simulink model "INDI_QUAD_2021a"  (R2026a)
settings: Solver=VariableStepAuto  StopTime=30  FixedStep=step_time
InitFcn:
  | kt = 66.34;
  | kq = 2.38;
  | M = 8.22;
  | l = 1.63/2;
  | Ix = 0.4688;
  | Iy = 0.5;
  | Iz = 0.4930;
  | g = 9.81;
  | step_time = 0.001;
  | Kz = 125;
  | Kpsi = 70;
  | Kphi = 70;
  | Ktheta = 70;
  | flt = 0.45;
undefined symbols (not defined in the file): F, Light, MIL
libraries: aerolibwind2 x1, sim3dlib x1, uavsim3dlib x1
settings Model: Creator=Lenovo  LastModifiedBy=Lenovo
settings SimscapeCC: SimscapeNominalValues="[{\"value\":\"1\",\"unit\":\"A\"},{\"value\":\"1\",\"unit\":\"bar\"},{\"value\":\"1\",\"unit\":\"cm^2\"},{\"value\":\"1\",\"unit\":\"cm^3/s\"},{\"value\":\"1\",\"unit\":\"kJ/kg\"},{\"value\":\"1\",\"unit\":\"kW\"},{\"value\":\"1\",\"unit\":\"l\"},{\"value\":\"1\",\"unit\":\"N\"},{\"value\":\"1\",\"unit\":\"N*m\"},{\"value\":\"1\",\"unit\":\"V\"}]"  SimscapeLogType=none  SimscapeLogDataHistory=5000.0

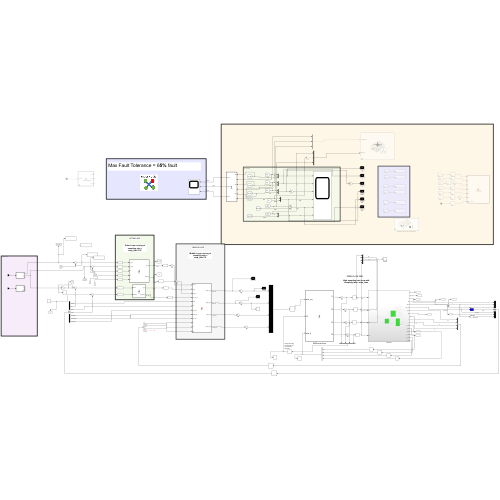
[thumbnail: Simulink's stored preview of the top-level diagram]
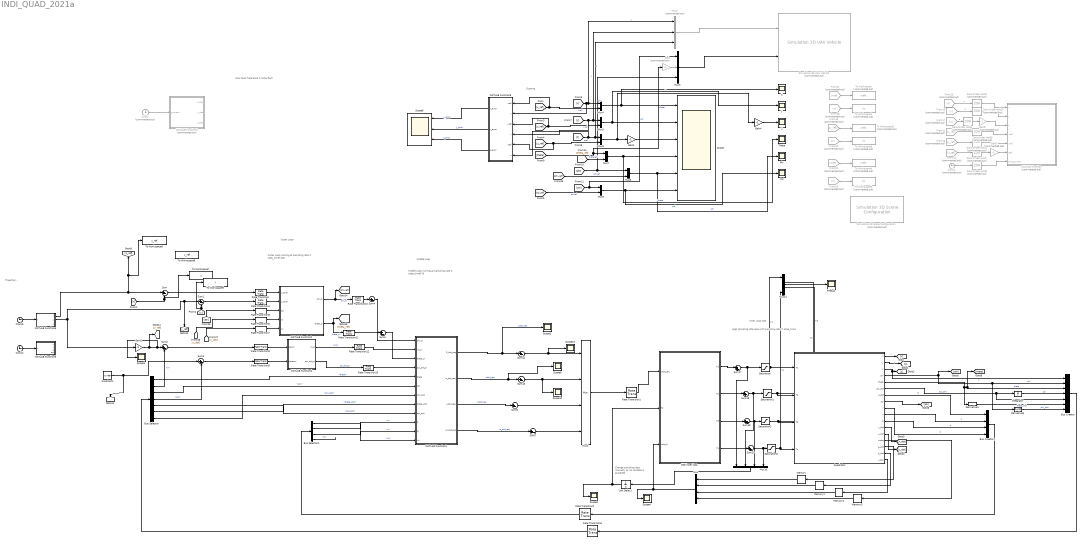
== system INDI_QUAD_2021a ==
  note: Inner Loop INDI
  note: Outer Loop
  note: Middle Loop running at sampling rate = step_time*10
  note: Trajectory
  note: Change sampling rate manually as no variable is assigned
  note: High sampling rate loop with sampling rate = step_time
  note: Max Fault Tolerance = 6 5% fault
  note: Outer Loop running at sampling rate = step_time*100
  note: Middle Loop
  note: Scoping
  Bus Creator : BusCreator  Inputs=7
  Bus Creator1 : BusCreator  Inputs=4
  Bus Selector : BusSelector  OutputSignals=theta,z,phi,psi,psi_dot,theta_dot,phi_dot
  Bus Selector1 : BusSelector  OutputSignals=Vz,p,q,R
  Clock : Clock  Commented=on
  Clock1 : Clock  Commented=on
  Clock2 : Clock
  Clock5 : Clock
  Constant1 : Constant  Value=0.7854
  Derivative1 : Derivative
  Derivative2 : Derivative
  From12 : From  Commented=on  GotoTag=x_ref
  From13 : From  Commented=on  GotoTag=y_ref
  From14 : From  Commented=on  GotoTag=z_ref
  From15 : From  Commented=on  GotoTag=x
  From16 : From  Commented=on  GotoTag=y
  From17 : From  Commented=on  GotoTag=z
  From18 : From  Commented=on  GotoTag=x
  From19 : From  Commented=on  GotoTag=y_ref
  From20 : From  Commented=on  GotoTag=zref
  From21 : From  Commented=on  GotoTag=xref
  From22 : From  Commented=on  GotoTag=y
  From23 : From  Commented=on  GotoTag=z
  Gain : Gain  Commented=on  Gain=-1
  Gain1 : Gain  Gain=-1
  Gain2 : Gain  Gain=-1
  Gain3 : Gain  Commented=on  Gain=-1
  Gain4 : Gain  Gain=-1
  Gain8 : Gain  Commented=on  Gain=-1
  INDI inner loop : MATLAB Function  TreatAsAtomicUnit=on
  Integrator : Integrator  InitialCondition=0.7854
  MATLAB Function : MATLAB Function  Commented=on  TreatAsAtomicUnit=on
  MATLAB Function1 : MATLAB Function  TreatAsAtomicUnit=on
  MATLAB Function2 : MATLAB Function  TreatAsAtomicUnit=on
  MATLAB Function3 : MATLAB Function  Commented=on  TreatAsAtomicUnit=on
  MATLAB Function4 : MATLAB Function  TreatAsAtomicUnit=on
  MATLAB Function5 : MATLAB Function  TreatAsAtomicUnit=on
  MATLAB Function6 : MATLAB Function  TreatAsAtomicUnit=on
  MATLAB Function8 : MATLAB Function  TreatAsAtomicUnit=on
  Memory{,1..3} (4 alike) : Memory
  Mux{,1,10..11} (4 alike) : Mux
  Mux2 : Mux  Commented=on  Inputs=3
  Mux3 : Mux  Inputs=3
  Mux{4..9} (6 alike) : Mux  Inputs=2
  Phi : Scope
      settings: Title=Roll angle (rad) vs Time (Seconds)  ActiveDisplayYMinimum=-0.24071  ActiveDisplayYMaximum=0.27138  YLabel=Roll angle (rad)
  Psi : Scope
      settings: Title=Yaw angle (rad) vs Time (Seconds)  ActiveDisplayYMinimum=-0.5  ActiveDisplayYMaximum=0.5  YLabel=Yaw angle (rad)  DataLoggingVariableName=ScopeData2
  Quadrotor : Subsystem
  Rate Transition{,4..9} (7 alike) : RateTransition  OutPortSampleTime=step_time*100
  Rate Transition1 : RateTransition  OutPortSampleTime=step_time
  Rate Transition{2..3,10..13} (6 alike) : RateTransition  OutPortSampleTime=step_time*10
  Saturation{,1..3} (4 alike) : Saturate  UpperLimit=1  LowerLimit=0
  Scope : Scope  NumInputPorts=6
      settings: TimeSpan=30  ActiveDisplayYMinimum=-1.4894  ActiveDisplayYMaximum=13.37546  YLabel=x(m)  DataLoggingVariableName=ScopeData3
  Scope{1..4,9,12..13} (7 alike) : Scope
      Scope1 settings: ActiveDisplayYMinimum=-11.25  ActiveDisplayYMaximum=1.25  DataLoggingVariableName=ScopeData3
      Scope12 settings: ActiveDisplayYMinimum=-0.77126  ActiveDisplayYMaximum=1.00462  DataLoggingVariableName=ScopeData5
      Scope13 settings: ActiveDisplayYMinimum=-0.61483  ActiveDisplayYMaximum=0.4623  DataLoggingVariableName=ScopeData6
      Scope2 settings: ActiveDisplayYMinimum=-0.24056  ActiveDisplayYMaximum=0.09054
      Scope3 settings: ActiveDisplayYMinimum=-0.1115  ActiveDisplayYMaximum=1.0035  DataLoggingVariableName=ScopeData5
      Scope4 settings: ActiveDisplayYMinimum=-8.06418  ActiveDisplayYMaximum=11.79602  DataLoggingVariableName=ScopeData6
      Scope9 settings: ActiveDisplayYMinimum=-0.58145  ActiveDisplayYMaximum=0.65087  DataLoggingVariableName=ScopeData2
  Scope6 : Scope  NumInputPorts=3
      settings: ActiveDisplayYMinimum=-0.92421  ActiveDisplayYMaximum=8.31793
  Simulation 3D Scene Configuration : sim3dlib/Simulation 3D Scene Configuration  Priority=0  Commented=on  ProjectFormat=Unreal Executable  SceneDesc=US city block  ProjectName=C:\Program Files\MATLAB\R2024a\toolbox\shared\sim3d_projects\automotive_project_windows\UE\WindowsNoEditor\VehicleSimulation.exe  ScenePath=/Game/Maps/USCityBlock  EnableOpenDRIVE=off  vehTagList={'Scene Origin'}  vehTag=Scene Origin  AttachedCameraRelativeTranslation=[0 0 0]  FreeCameraDefaultInitialTranslation=[-6, 0, 2]  AttachedCameraRelativeRotation=[0, -15, 0]  FreeCameraDefaultInitialRotation=[0, -15, 0]  ViewpointName=Custom  FreeCameraInitialTranslation=[0, 0, 0]  FreeCameraInitialRotation=[0, 0, 0]  OpVisEn=off  Ts=step_time*10  EnableWindow=on  EnableRemoteAccess=off  SimulationMode=CoSimulation  SimulateUsing=Interpreted execution  EnableAnimationRecording=off  OverrideDefaultRecording=off  AnimationRecordingFileName=sim3dAnimation.mat  AnimationRecordingInterval=[0 inf]  EnableWeather=off  SunAzimuth=90  SunAltitude=40.0  EnableGeospatialSun=off  Latitude=0  Longitude=0  Date=2023-01-01  Time=10:30:00  GeoTimeZone=-5.0  SunDaylightSaving=off  wind=1  clouds=10  EnableVolumetricClouds=off  CloudCoverage=0  CloudAltitude=6  fog=0  rain=0  RaindropsEffect=off  SnowDensity=0  EnableGeospatial=off  TilesetSource=Earth terrain  UseTrueOrigin=off  OriginHeight=200  OriginLatitude=40.744652  OriginLongitude=-73.988864  MapStyle=Aerial  AdditionalAssetIDs=[]  UseAdvancedSunSky=off  SolarTime=11  TimeZone=-5  Day=21  Month=9  Year=2022  UseDaylightSavingTime=on  DSTStartDay=10  DSTStartMonth=3  DSTEndDay=3  DSTEndMonth=11  DSTSwitchHour=2  sensorTag=MainCamera1  sensorId=1  sensorName=MainCamera1  mountLoc=Origin  offsetFlag=off  tmountOffset=[0, 0, 0]  rmountOffset=[0, 0, 0]  HorizontalResolution=1280  VerticalResolution=720  HorizontalFOV=60  mountPoint=[0 0 0]  mountOrientation=[0 0 0]  aMode=4  ID=1  GeoTrigger=Inactive  ViewNameList={'Custom'}  ViewTranslationList={'[0 0 0]'}  ViewRotationList={'[0 0 0]'}
      settings: LibrarySourceBlock=uavsim3dlib/Simulation 3D Scene Configuration
  Simulation 3D UAV Vehicle : uavsim3dlib/Simulation 3D UAV Vehicle  Priority=-1  Commented=on  Mesh=Quadrotor  MeshPath=/MathWorksUAVContent/UAVs/HexaRotorUAV/HexaRotor.HexaRotor  Color=Black  ActorName=SimulinkVehicle1  UseGlobalFrame=off  InitialTranslation=[0 0 0]  InitialRotation=[0 0 0]  InitialTranslationGlobal=[0 0 0]  InitialGeoOrigin=[0 0 0]  InitialRotationGlobal=[0 0 0]  SampleTime=-1  ActorType=SimulinkVehicle  ID=1  aMode=4  ActorTag=SimulinkVehicle1
  Sum{,1..7,13..14} (10 alike) : Sum  Inputs=|+-
  Sum{17..20} (4 alike) : Sum  Inputs=|++
  THeta : Scope
      settings: Title=Pitch angle (rad) vs Time (Seconds)  ActiveDisplayYMinimum=-0.27265  ActiveDisplayYMaximum=0.23706  YLabel=Pitch angle (rad)  DataLoggingVariableName=ScopeData4
  THeta1 : Scope
      settings: Title=Normalized Thrust Force vs Time (seconds)  ActiveDisplayYMinimum=-0.11657  ActiveDisplayYMaximum=1.04914  YLabel=Normalized Thrust Force  DataLoggingVariableName=ScopeData2
  To Workspace : ToWorkspace  Commented=on  VariableName=xreflc  SampleTime=-1
  To Workspace1 : ToWorkspace  Commented=on  VariableName=xlc  SampleTime=-1
  To Workspace2 : ToWorkspace  Commented=on  VariableName=yreflc  SampleTime=-1
  To Workspace3 : ToWorkspace  Commented=on  VariableName=ylc  SampleTime=-1
  To Workspace4 : ToWorkspace  Commented=on  VariableName=zreflc  SampleTime=-1
  To Workspace5 : ToWorkspace  Commented=on  VariableName=zlc  SampleTime=-1
  To Workspace6 : ToWorkspace  VariableName=x_ref  SaveFormat=Timeseries  SampleTime=-1
  To Workspace7 : ToWorkspace  VariableName=x  SaveFormat=Timeseries  SampleTime=-1
  To Workspace8 : ToWorkspace  VariableName=y_ref  SaveFormat=Timeseries  SampleTime=-1
  To Workspace9 : ToWorkspace  VariableName=y  SaveFormat=Timeseries  SampleTime=-1
  Unit Delay1 : UnitDelay  SampleTime=step_time
  X : Scope
      settings: Title=x (m) vs Time (Seconds)  ActiveDisplayYMinimum=-1.43359  ActiveDisplayYMaximum=12.90232  YLabel=X(m)  DataLoggingVariableName=ScopeData5
  Y : Scope
      settings: Title=y (m) vs Time (Seconds)  ActiveDisplayYMinimum=-1.44356  ActiveDisplayYMaximum=12.99204  YLabel=y(m)  DataLoggingVariableName=ScopeData6
  Z : Scope
      settings: Title=z (m) vs Time (Seconds)  ActiveDisplayYMinimum=-1.37451  ActiveDisplayYMaximum=12.30742  YLabel=z(m)  DataLoggingVariableName=ScopeData7
  Zero-Order Hold{2..8} (7 alike) : ZeroOrderHold  Commented=on  SampleTime=0.1
  wires:
  Bus Creator1/1 -> Rate Transition2/1
  Quadrotor/5(theta) -> Bus Creator/3, [theta], Derivative1/1  "theta"
  Quadrotor/4(phi) -> Derivative2/1, Bus Creator/2, [phi]  "phi"
  Quadrotor/2(y) -> [y]  "y"
  Quadrotor/6(psi_dot) -> Bus Creator/5, Integrator/1  "psi_dot"
  Quadrotor/3(z) -> Bus Creator/1, [z]  "z"
  Quadrotor/1(x) -> [x]  "x"
  Quadrotor/11(q) -> Bus Creator1/3  "q"
  Quadrotor/14(vzdot) -> Memory3/1
  Bus Creator/1 -> Rate Transition3/1
  Quadrotor/8(psi) -> [psi]
  Quadrotor/12(x_dot) -> [x_dot]
  Quadrotor/10(p) -> Bus Creator1/2  "p"
  Quadrotor/13(y_dot) -> [y_dot]
  Quadrotor/7(z_dot) -> Bus Creator1/1  "Vz"
  Quadrotor/9(r) -> Bus Creator1/4  "R"
  Integrator/1 -> Bus Creator/4  "psi"
  Bus Selector/3 -> MATLAB Function1/6(phi)  "<phi>"
  Bus Selector/1 -> MATLAB Function1/5(theta)  "<theta>"
  Derivative1/1 -> Bus Creator/6  "theta_dot"
  Derivative2/1 -> Bus Creator/7  "phi_dot"
  Bus Selector/5 -> MATLAB Function1/9(psi_dot)  "<psi_dot>"
  Bus Selector/6 -> MATLAB Function1/8(theta_dot)  "<theta_dot>"
  Bus Selector/7 -> MATLAB Function1/7(phi_dot)  "<phi_dot>"
  Bus Selector1/1 -> MATLAB Function1/12(Vz)  "<Vz>"
  Bus Selector1/2 -> MATLAB Function1/10(P)  "<p>"
  Bus Selector1/3 -> MATLAB Function1/11(Q)  "<q>"
  Bus Selector1/4 -> ?  "<R>"
  Rate Transition2/1 -> Bus Selector1/1
  Rate Transition3/1 -> Bus Selector/1
  Clock/1 -> MATLAB Function3/1(t_current)
  Mux10/1 -> Unit Delay1/1
  Mux1/1 -> Rate Transition1/1
  Rate Transition1/1 -> INDI inner loop/1(xdot_req)
  Memory/1 -> Mux/1
  Memory1/1 -> Mux/2
  Memory2/1 -> Mux/3
  Memory3/1 -> Mux/4
  Bus Selector/4 -> Sum3/2  "<psi>"
  Sum1/1 -> Rate Transition4/1
  Sum/1 -> Rate Transition/1
  Bus Selector/2 -> Sum2/2  "<z>"
  [x] -> To Workspace7/1, Sum/2
  [y] -> To Workspace9/1, Sum1/2
  Clock5/1 -> MATLAB Function6/1(t)
  MATLAB Function4/2(psi_dot_d) -> Rate Transition13/1  "psi_dot_d"
  MATLAB Function1/4(vz_dot_req) -> Sum7/1  "vz_dot_req"
  Mux/1 -> Scope4/1, INDI inner loop/3(xdot_0)
  MATLAB Function1/1(P_dot_req) -> Scope2/1, Sum14/1  "pdot_req"
  MATLAB Function1/2(q_dot_req) -> Scope9/1, Sum13/1  "qdot_req"
  Sum2/1 -> Rate Transition9/1
  MATLAB Function4/1(vz_d) -> Rate Transition12/1  "vz_d"
  MATLAB Function1/3(r_dot_req) -> Sum6/1  "r_dot_req"
  [x_dot] -> Rate Transition7/1
  Sum3/1 -> Rate Transition5/1
  MATLAB Function2/1(phi_d) -> [phi_ref], Rate Transition10/1  "phi_d"
  MATLAB Function2/2(theta_d) -> [theta_ref], Rate Transition11/1  "theta_d"
  Rate Transition/1 -> MATLAB Function2/1(x_error)
  Rate Transition4/1 -> MATLAB Function2/2(y_error)
  [psi] -> Rate Transition8/1
  [y_dot] -> Rate Transition6/1
  Rate Transition8/1 -> MATLAB Function2/3(psi)
  Rate Transition9/1 -> MATLAB Function4/1(zerror)
  Rate Transition5/1 -> MATLAB Function4/2(psierror)
  Rate Transition6/1 -> MATLAB Function2/4(Vy)
  Rate Transition7/1 -> MATLAB Function2/5(Vx)
  Mux5/1 -> Y/1, Scope/2  "y"
  [psi_ref] -> Mux9/2  "psiref"
  [y_ref] -> MATLAB Function8/3(yref), Mux5/2  "yref"
  Gain1/1 -> Scope/3
  [theta_ref] -> Mux7/2  "thetaref"
  Mux8/1 -> Phi/1, Scope/5  "phi"
  [z_ref] -> MATLAB Function8/5(zref), Mux6/2  "zref"
  [phi_ref] -> Mux8/2  "phiref"
  From19/1 -> To Workspace2/1
  [x_ref] -> MATLAB Function8/1(xref), Mux4/2  "xref"
  From21/1 -> To Workspace/1
  From18/1 -> To Workspace1/1
  Gain/1 -> Mux3/2
  [theta] -> Mux7/1, Gain/1  "theta"
  From20/1 -> To Workspace4/1
  Mux2/1 -> Simulation 3D UAV Vehicle/1
  Mux6/1 -> Gain4/1, Gain1/1
  Mux3/1 -> Simulation 3D UAV Vehicle/2
  From23/1 -> To Workspace5/1
  [z] -> MATLAB Function8/6(z), Mux2/3, Mux6/1  "z"
  [psi] -> Mux3/1, Mux9/1  "psi"
  Mux9/1 -> Psi/1, Scope/6  "psi"
  [phi] -> Mux8/1, Mux3/3  "phi"
  From22/1 -> To Workspace3/1
  Mux4/1 -> X/1, Scope/1
  Mux7/1 -> THeta/1, Scope/4  "theta"
  [x] -> MATLAB Function8/2(x), Mux2/1, Mux4/1  "x"
  [y] -> MATLAB Function8/4(y), Mux2/2, Mux5/1  "y"
  Clock1/1 -> Zero-Order Hold8/1
  Zero-Order Hold7/1 -> Gain3/1
  Gain8/1 -> MATLAB Function/3(z)
  Zero-Order Hold3/1 -> MATLAB Function/2(y)
  Zero-Order Hold8/1 -> MATLAB Function/7(time_current)
  Zero-Order Hold5/1 -> MATLAB Function/4(xref)
  From15/1 -> Zero-Order Hold2/1  "x"
  Zero-Order Hold4/1 -> Gain8/1
  From14/1 -> Zero-Order Hold7/1
  Zero-Order Hold6/1 -> MATLAB Function/5(yref)
  From12/1 -> Zero-Order Hold5/1
  From17/1 -> Zero-Order Hold4/1  "z"
  Zero-Order Hold2/1 -> MATLAB Function/1(x)
  From13/1 -> Zero-Order Hold6/1
  From16/1 -> Zero-Order Hold3/1  "x"
  Saturation/1 -> Mux11/1, Quadrotor/1(T1)  "T1"
  Saturation1/1 -> Mux11/2, Quadrotor/2(T2)  "T2"
  Saturation2/1 -> Mux11/3, Quadrotor/3(T3)  "T3"
  Clock2/1 -> MATLAB Function5/1(t)
  Gain2/1 -> [z_ref], Scope1/1, Sum2/1
  Gain3/1 -> MATLAB Function/6(zref)
  Quadrotor/16(q_dot) -> Memory1/1
  Quadrotor/17(r_dot) -> Memory2/1
  Quadrotor/15(p_dot) -> Memory/1
  Gain4/1 -> Z/1
  Mux11/1 -> THeta1/1
  Saturation3/1 -> Mux11/4, Quadrotor/4(T4)  "T4"
  MATLAB Function6/1(x) -> Sum/1, To Workspace6/1, [x_ref]
  Unit Delay1/1 -> Scope3/1, INDI inner loop/2(T0)
  Rate Transition10/1 -> Sum4/1
  Rate Transition11/1 -> Sum5/1
  Rate Transition12/1 -> MATLAB Function1/2(Vz_d)
  Sum4/1 -> MATLAB Function1/1(phi_d)
  Sum5/1 -> MATLAB Function1/3(theta_d)
  Rate Transition13/1 -> MATLAB Function1/4(psi_dot_d)
  Constant1/1 -> [psi_ref], Sum3/1
  Sum13/1 -> Scope12/1, Mux1/2
  Sum14/1 -> Scope13/1, Mux1/1
  Sum6/1 -> Mux1/3
  Sum7/1 -> Mux1/4
  MATLAB Function6/2(y) -> [y_ref], Sum1/1, Gain2/1
  MATLAB Function8/1(x_error) -> Scope6/1  "x_error"
  MATLAB Function8/2(y_error) -> Scope6/2  "y_error"
  MATLAB Function8/3(z_error) -> Scope6/3  "z_error"
  INDI inner loop/1(T1) -> Sum17/1
  Sum17/1 -> Mux10/1, Saturation/1
  INDI inner loop/2(T2) -> Sum18/1
  Sum19/1 -> Saturation2/1, Mux10/3
  INDI inner loop/3(T3) -> Sum19/1
  Sum20/1 -> Mux10/4, Saturation3/1
  INDI inner loop/4(T4) -> Sum20/1
  Sum18/1 -> Mux10/2, Saturation1/1

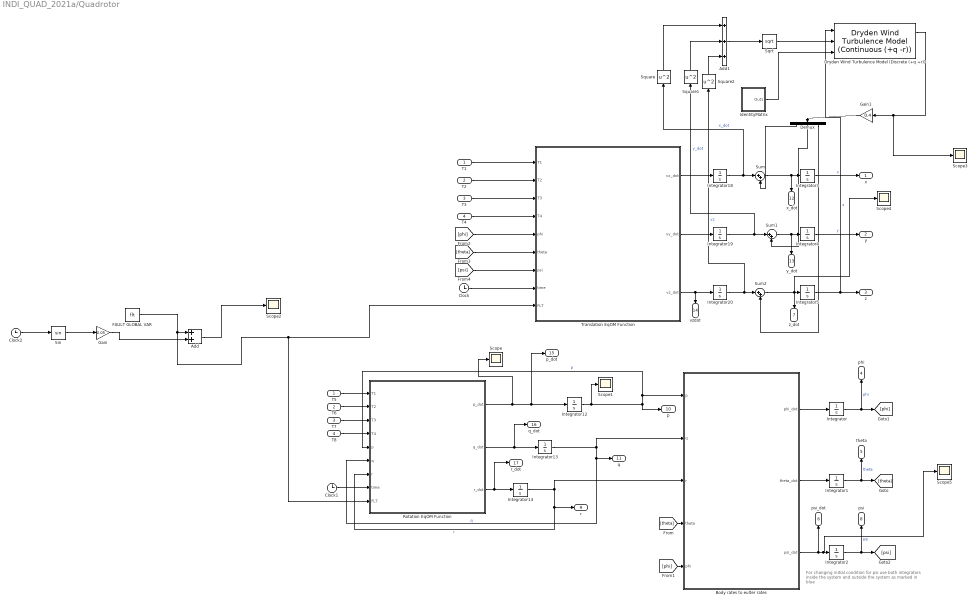
== system INDI_QUAD_2021a/Quadrotor ==
  note: For changing initial condition for psi use both integrators inside the system and outside the system as marked in blue
  T1 : Inport
  T2 : Inport  Port=2
  T3 : Inport  Port=3
  T4 : Inport  Port=4
  Add : Sum
  Add1 : Sum  Inputs=+++
  Body rates to eulter rates : MATLAB Function  TreatAsAtomicUnit=on
  Clock : Clock
  Clock1 : Clock
  Clock2 : Clock
  Demux : Demux  Outputs=3
  Dryden Wind Turbulence Model (Discrete (+q +r)) : aerolibwind2/Dryden Wind Turbulence Model  (Continuous (+q -r))  units=Metric (MKS)  spec=MIL-F-8785C  model=Discrete Dryden (+q +r)  W20=15  Wdeg=0  TurbProb=10^-2 - Light  L_high=533.4  Wingspan=10  ts=0.1  Seed=[23341 23342 23343 23344]  T_on=on
  FAULT GLOBAL VAR : Constant  Value=flt
  Gain : Gain  Gain=0.05
  Gain1 : Gain  Gain=0.4
  IdentityMatrix : Subsystem  Description=Replaced Block  mask(Replaced Block){}
      mask help: This block has been replaced with an empty subsystem because it used functionality that is unavailable in Simulink R2021a.
      mask Display: fprintf('Replaced: %s\n','IdentityMatrix')
  Integrator : Integrator  WrapState=on
  Integrator1 : Integrator  WrapState=on
  Integrator{3..5,12..14,18..20} (9 alike) : Integrator
  Integrator2 : Integrator  InitialCondition=0.7854  WrapState=on
  Rotation EqOM Function : MATLAB Function  TreatAsAtomicUnit=on
  Scope{,1..5} (6 alike) : Scope
      Scope settings: ActiveDisplayYMinimum=-4.36641  ActiveDisplayYMaximum=4.97625  DataLoggingVariableName=ScopeData2
      Scope1 settings: ActiveDisplayYMinimum=-0.32703  ActiveDisplayYMaximum=0.13523  DataLoggingVariableName=ScopeData3
      Scope2 settings: ActiveDisplayYMinimum=0.3875  ActiveDisplayYMaximum=0.5125
      Scope3 settings: ActiveDisplayYMinimum=-4.66573  ActiveDisplayYMaximum=4.5685
      Scope4 settings: ActiveDisplayYMinimum=-7.86748  ActiveDisplayYMaximum=3.63162  DataLoggingVariableName=ScopeData5
      Scope5 settings: ActiveDisplayYMinimum=-0.04461  ActiveDisplayYMaximum=0.03015  DataLoggingVariableName=ScopeData6
  Sin : Trigonometry
  Sqrt : Sqrt
  Square : Math  Operator=square
  Square1 : Math  Operator=square
  Square2 : Math  Operator=square
  Sum : Sum  Inputs=|++
  Sum1 : Sum  Inputs=|++
  Sum2 : Sum  Inputs=|++
  T5 : InportShadow
  T6 : InportShadow  Port=2
  T7 : InportShadow  Port=3
  T8 : InportShadow  Port=4
  Translation EqOM Function : MATLAB Function  TreatAsAtomicUnit=on
  x : Outport
  y : Outport  Port=2
  z : Outport  Port=3
  phi : Outport  Port=4
  theta : Outport  Port=5
  psi_dot : Outport  Port=6
  z_dot : Outport  Port=7
  psi : Outport  Port=8
  r : Outport  Port=9
  p : Outport  Port=10
  q : Outport  Port=11
  x_dot : Outport  Port=12
  y_dot : Outport  Port=13
  vzdot : Outport  Port=14
  p_dot : Outport  Port=15
  q_dot : Outport  Port=16
  r_dot : Outport  Port=17
  wires:
  [phi] -> Body rates to eulter rates/5(phi)
  T8/1 -> Rotation EqOM Function/4(T4)
  Rotation EqOM Function/3(r_dot) -> r_dot/1, Integrator14/1
  Integrator18/1 -> Sum/1, Square/1  "x_dot"
  [theta] -> Translation EqOM Function/6(theta)
  Integrator14/1 -> Body rates to eulter rates/3(r), r/1, Rotation EqOM Function/7(r)  "r"
  Integrator20/1 -> Sum2/1, Square2/1  "vz"
  Integrator12/1 -> Scope1/1, Rotation EqOM Function/5(p), Body rates to eulter rates/1(p), p/1  "p"
  Translation EqOM Function/2(vy_dot) -> Integrator19/1
  Integrator13/1 -> Body rates to eulter rates/2(q), q/1, Rotation EqOM Function/6(q)  "q"
  Integrator1/1 -> theta/1, [theta]  "theta"
  Translation EqOM Function/3(vz_dot) -> vzdot/1, Integrator20/1
  Integrator/1 -> phi/1, [phi]  "phi"
  [theta] -> Body rates to eulter rates/4(theta)
  Rotation EqOM Function/1(p_dot) -> Scope/1, p_dot/1, Integrator12/1
  Rotation EqOM Function/2(q_dot) -> q_dot/1, Integrator13/1
  T4/1 -> Translation EqOM Function/4(T4)
  Integrator19/1 -> Sum1/1, Square1/1  "y_dot"
  Translation EqOM Function/1(vx_dot) -> Integrator18/1
  Integrator2/1 -> psi/1, [psi]  "psi"
  T7/1 -> Rotation EqOM Function/3(T3)
  T3/1 -> Translation EqOM Function/3(T3)
  Body rates to eulter rates/1(phi_dot) -> Integrator/1
  T1/1 -> Translation EqOM Function/1(T1)
  [phi] -> Translation EqOM Function/5(phi)
  Body rates to eulter rates/2(theta_dot) -> Integrator1/1
  [psi] -> Translation EqOM Function/7(psi)
  T6/1 -> Rotation EqOM Function/2(T2)
  T2/1 -> Translation EqOM Function/2(T2)
  T5/1 -> Rotation EqOM Function/1(T1)
  Integrator3/1 -> x/1  "x"
  Integrator4/1 -> y/1  "y"
  Integrator5/1 -> Dryden Wind Turbulence Model (Discrete (+q +r))/1, z/1  "z"
  Clock/1 -> Translation EqOM Function/8(time)
  Clock1/1 -> Rotation EqOM Function/8(time)
  Sin/1 -> Gain/1
  Clock2/1 -> Sin/1
  Gain/1 -> Add/2
  FAULT GLOBAL VAR/1 -> Add/1, Rotation EqOM Function/9(FLT), Translation EqOM Function/9(FLT)
  IdentityMatrix/1(Out1) -> Dryden Wind Turbulence Model (Discrete (+q +r))/3
  Add1/1 -> Sqrt/1
  Sqrt/1 -> Dryden Wind Turbulence Model (Discrete (+q +r))/2
  Square/1 -> Add1/1
  Square1/1 -> Add1/2
  Square2/1 -> Add1/3
  Dryden Wind Turbulence Model (Discrete (+q +r))/1 -> Scope3/1, Gain1/1
  Sum/1 -> x_dot/1, Integrator3/1
  Demux/1 -> Sum/2
  Sum1/1 -> y_dot/1, Integrator4/1
  Demux/2 -> Sum1/2
  Demux/3 -> Sum2/2
  Gain1/1 -> Demux/1
  Sum2/1 -> z_dot/1, Scope4/1, Integrator5/1
  Body rates to eulter rates/3(psi_dot) -> psi_dot/1, Scope5/1, Integrator2/1
  Add/1 -> Scope2/1

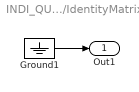
== system INDI_QUAD_2021a/Quadrotor/IdentityMatrix ==
  Ground1 : Ground
  Out1 : Outport
  wires:
  Ground1/1 -> Out1/1

== matlab function INDI_QUAD_2021a/Quadrotor/Translation EqOM Function ==
  data: T1 input; vx_dot output; T2 input; T3 input; T4 input; phi input; theta input; psi input; vy_dot output; vz_dot output; time input; FLT input
function [vx_dot, vy_dot,vz_dot] = fcn(T1,T2,T3,T4,phi,theta,psi,time,FLT)
kt = 66.34;
kq = 2.3114; 
M = 8.22;
l = 1.83/2;
Ix = 0.4688;
Iy = 0.7639;
Iz = 0.4930;
g = 9.81;
    if (time>7.5)
        fault = FLT;
    else
        fault = 1;
    end


    A = (sin(phi)*sin(psi)+cos(phi)*sin(theta)*cos(psi));
    B = (-sin(phi)*cos(psi) + cos(phi)*sin(theta)*sin(psi));
    C = (cos(phi)*cos(theta));

    GX = [-fault*(A/M)*kt,-(A/M)*kt,-(A/M)*kt,-(A/M)*kt;
        -fault*(B/M)*kt,-(B/M)*kt,-(B/M)*kt,-(B/M)*kt;
        -fault*(C/M)*kt,-(C/M)*kt,-(C/M)*kt,-(C/M)*kt;];

    Tx = [T1;T2;T3;T4];
    fx = [0;0;g];
        
    linear_accel = GX*Tx +fx;

    vx_dot = linear_accel(1);
    vy_dot = linear_accel(2);
    vz_dot = linear_accel(3);

== matlab function INDI_QUAD_2021a/MATLAB Function4 ==
  data: zerror input; vz_d output; psierror input; psi_dot_d output
function [vz_d, psi_dot_d]= fcn(zerror,psierror)

Kz =5;
Kpsi = 2.5;

Error = [zerror;psierror];
Gain = [Kz 0;
    0 Kpsi];

out = Gain*Error;

vz_d = out(1);
psi_dot_d = out(2);

end

== matlab function INDI_QUAD_2021a/MATLAB Function5 ==
  data: x output; y output; z output; psi output; t input
function [x, y, z, psi] = fcn(t)
% fcn - Generates a smooth helical trajectory starting and ending at the origin
% Inputs:
%   t   - simulation time [s]
% Outputs:
%   x, y, z - position coordinates
%   psi     - yaw angle (rad)

% Parameters
t_up = 50;                      % Ascent duration (s)
t_total = 60;                   % Total simulation time (s)
R = 5;                          % Radius of helix
h = 10;                         % Max height
n_turns = 3;                    % Helix turns
omega = 2 * pi * n_turns / t_up;  % Angular speed

% Initialize outputs
x = 0; y = 0; z = 0; psi = 0;

if t <= t_up
    % Ascent phase
    x = R * sin(omega * t);
    y = R * (1 - cos(omega * t));   % starts at y = 0
    z = h * t / t_up;
    psi = mod(omega * t, 2*pi);

elseif t > t_up && t <= t_total
    % Return phase
    tau = (t - t_up) / (t_total - t_up);  % Normalized time [0, 1]

    % Position at top (t = 50)
    x0 = R * sin(omega * t_up);
    y0 = R * (1 - cos(omega * t_up));
    z0 = h;
    psi0 = mod(omega * t_up, 2*pi);

    % Smoothstep interpolation (cubic)
    s = 1 - 3*tau^2 + 2*tau^3;

    x = x0 * s;
    y = y0 * s;
    z = z0 * s;
    psi = psi0 * s;

else
    % Post-landing: stay at origin
    x = 0;
    y = 0;
    z = 0;
    psi = 0;
end

end

== matlab function INDI_QUAD_2021a/MATLAB Function6 ==
  data: x output; t input; y output; z output
function [x, y, z] = fcn(t)
    if t < 1
        x = 0;
        y = 0;
        z = 0;

    elseif t >= 1 && t < 15
        x = 10 * tanh(0.6 * (t - 1));
        y = 10 * tanh(0.6 * (t - 1));

        % Corrected parabolic z trajectory: peak at t=7.5, z=10; z=0 at t=1 and t=14
        a = -10 / (7.5 - 1)^2;
        z = a * (t - 7.5)^2 + 10;

    else
        x = 10 * tanh(0.6 * (t - 1));
        y = 10 * tanh(0.6 * (t - 1));
        z = 0;
    end
end

== matlab function INDI_QUAD_2021a/MATLAB Function8 ==
  settings: updateMethod=DISCRETE
  data: xref input; x_error output; x input; yref input; y input; zref input; z input; y_error output; z_error output
function [x_error,y_error,z_error] = fcn(xref, x,yref,y,zref,z)
    x_error = abs(x-xref);
    y_error = abs(y-yref);
    z_error = abs(z-zref);
end

== matlab function INDI_QUAD_2021a/MATLAB Function ==
  settings: updateMethod=DISCRETE
  data: x input; y input; z input; xref input; yref input; zref input; time_current input
function plotTrajectory(x, y, z, xref, yref, zref,time_current)
    %#codegen
    persistent h;  % Use persistent to keep the figure window open.
    persistent xHistory yHistory zHistory;  % Store history of actual positions
    persistent xrefHistory yrefHistory zrefHistory;  % Store history of reference positions
    
    if isempty(h)
        h = figure;  % Create a figure window if it doesn't exist.
        xHistory = [];  % Initialize history arrays
        yHistory = [];
        zHistory = [];
        xrefHistory = [];  % Initialize reference history arrays
        yrefHistory = [];
        zrefHistory = [];
    end

    % Update the history with the current position
    xHistory = [xHistory; x];  % Append current x
    yHistory = [yHistory; y];  % Append current y
    zHistory = [zHistory; z];  % Append current z

    % Update the history with the reference position
    xrefHistory = [xrefHistory; xref];  % Append current xref
    yrefHistory = [yrefHistory; yref];  % Append current yref
    zrefHistory = [zrefHistory; zref];  % Append current zref

    % Open the existing figure window and clear it for fresh plotting.
    figure(h);
    clf;  % Clear the current figure to prevent overlapping plots.

    % Plot the historical actual trajectory with a solid blue line.
    plot3(xHistory, yHistory, zHistory, 'k-', 'LineWidth', 2);  % Historical trajectory
    hold on;
    if abs(time_current - 15) < 1  % Check if we're at t = 15 seconds (allowing a small tolerance)
        plot3(x, y, z, 'bo', 'MarkerSize', 12, 'LineWidth', 2);  % Larger blue circle
    end
    hold on;
    % Plot the historical reference trajectory with a dashed red line.
    plot3(xrefHistory, yrefHistory, zrefHistory, 'r--', 'LineWidth', 2);  % Reference trajectory
    
    hold on;

    % Labels for clarity.
    xlabel('X Axis');
    ylabel('Y Axis');
    zlabel('Z Axis');
    grid on;

    % Set fixed axis limits from -10 to 30 for x and y, and 0 to 30 for z.
    xlim([0, 20]);  % Set X limits
    ylim([0, 20]);  % Set Y limits
    zlim([0, 20]);  % Set Z limits

    % Ensure the axes are orthogonal by enforcing a 1:1:1 aspect ratio.
    daspect([1 1 1]);

    % Set the viewing angle for a clear 3D perspective.
    view(3);

    % Add a legend to differentiate actual and reference trajectories.
    legend('Actual Trajectory', 'Reference Trajectory', 'Reference Trajectory');

    % Keep hold on for further updates.
    hold off;
end

== matlab function INDI_QUAD_2021a/MATLAB Function3 ==
  data: x_des output; t_current input; y_des output; z_des output
function [x_des, y_des, z_des] = trajectory_generator(t_current)
    % TRAJECTORY_GENERATOR Function to provide desired x, y, z values 
    % for the specified mission profile with a circular path centered at (2.5, 2.5, 10).
    % Input:
    %   t_current: Current time in simulation (seconds)
    % Outputs:
    %   x_des: Desired x position at time t_current
    %   y_des: Desired y position at time t_current
    %   z_des: Desired z position at time t_current

    % Mission profile parameters
    total_time = 50;    % Total simulation time (seconds)
    radius = 8;         % Radius of the circular path (in meters)
    z_takeoff = 10;     % Height of takeoff and final hover (in meters)
    circle_center_x = radius*cos(pi/4); % X-coordinate of the circle center
    circle_center_y = radius*sin(pi/4); % Y-coordinate of the circle center
    takeoff_time = 10;  % Time for takeoff (in seconds)
    circle_time = 30;   % Time to complete the circular motion (in seconds)
    landing_time = 10;  % Time for landing (in seconds)

    % Initialize the desired positions
    x_des = 0;
    y_des = 0;
    z_des = 0;

    % Phase 1: Takeoff (0 to 10 seconds)
    if t_current <= takeoff_time
        z_des = z_takeoff * (t_current / takeoff_time);  % Linear takeoff to 10m

    % Phase 2: Circular motion at z = 10m, centered at (2.5, 2.5) (10 to 30 seconds)
    elseif t_current > takeoff_time && t_current <= (takeoff_time + circle_time)
        % Calculate the angle for circular motion
        theta = 2 * pi * ((t_current - takeoff_time) / circle_time)+(225*(pi/180));
        x_des = circle_center_x + radius * cos(theta);  % Offset the circle center
        y_des = circle_center_y + radius * sin(theta);
        z_des = z_takeoff;  % Constant altitude during circular motion

    % Phase 3: Return to (0, 0, 10) and landing (30 to 40 seconds)
    elseif t_current > (takeoff_time + circle_time) && t_current <= total_time
        frac = (t_current - (takeoff_time + circle_time)) / landing_time;
        x_des = 0;  % Interpolate back to 0,0
        y_des = 0;
        z_des = z_takeoff * (1 - frac);  % Descend to 0 during landing

    % After total time, stay at origin (landed)
    else
        x_des = 0;
        y_des = 0;
        z_des = 0;
    end
end

== matlab function INDI_QUAD_2021a/Quadrotor/Body rates to eulter rates ==
  data: p input; phi_dot output; q input; r input; theta input; phi input; theta_dot output; psi_dot output
function [phi_dot,theta_dot,psi_dot] = fcn(p,q,r,theta,phi)
    R = [1, sin(phi)*tan(theta), cos(phi)*tan(theta);
        0, cos(phi), -sin(phi);
        0, sin(phi)/cos(theta), cos(phi)/cos(theta)];
    brates = [p;q;r];
    euler_rates = R*brates;
    phi_dot = euler_rates(1);
    theta_dot = euler_rates(2);
    psi_dot = euler_rates(3);

== matlab function INDI_QUAD_2021a/INDI inner loop ==
  data: xdot_req input; T0 input; xdot_0 input; T1 output; T2 output; T3 output; T4 output
function [T1, T2, T3, T4] = fcn(xdot_req,T0,xdot_0)

neta =1;

v = xdot_req;%from middle loop (Reference acceleration values)
ddx = xdot_0;%Previous time step value. (First term in Taylors series expansion).
T_0 = T0(:);

gx =neta*[-129.598,129.598,129.598,-129.598;
    79.534,-79.534,79.534,-79.534 ;
    4.6884,4.6884,-4.6884,-4.6884 ;
  -8.07785,-8.07785,-8.07785,-8.07785];%Changed according to new motor model specifications



gx_inv = inv(gx); %Inversion of control effectiveness matrix

diff = (v-ddx); % (v - xdot_0) in the control law.
dT = gx_inv*(diff);%multiplication with inverse of control effectiveness matrix.

T = dT +T_0; %Incrementing the delta_U with previous U_0 value to get the new U value.

T1 = T(1);
T2 = T(2);
T3 = T(3);
T4 = T(4);

== matlab function INDI_QUAD_2021a/MATLAB Function2 ==
  data: x_error input; phi_d output; y_error input; psi input; Vy input; Vx input; theta_d output
function [phi_d,theta_d] = fcn( x_error,y_error,psi,Vy,Vx)
K1x =0.0085;
K2x =0.014;
K3x =0.9;

K1y =0.00851;
K2y =0.014;
K3y =0.9000;
Error1 = [x_error; y_error];
Gain1 = [K1x 0;
    0 K1y];

V = Gain1*Error1;

Vx_d = V(1);
Vy_d = V(2);

Error2 = [(Vx_d - (K2x*Vx)); (Vy_d-(K2y*Vy))];
Gain2 = [K3x 0;
    0 K3y];

Act = Gain2*Error2;

Ax = Act(1);
Ay = Act(2);

A_f = Ax*(cos(psi))+Ay*(sin(psi));
A_r = -Ax*(sin(psi))+Ay*(cos(psi));

theta_d = (atan(-A_f/(9.81)))*180/pi;
phi_d = (atan((A_r*cos(theta_d))/(9.81))*180/pi);

end

== matlab function INDI_QUAD_2021a/MATLAB Function1 ==
  data: phi_d input; Vz_d input; theta_d input; psi_dot_d input; theta input; P_dot_req output; phi input; phi_dot input; theta_dot input; psi_dot input; P input; Q input; Vz input; q_dot_req output; r_dot_req output; vz_dot_req output
function [P_dot_req, q_dot_req, r_dot_req, vz_dot_req] = fcn(phi_d,Vz_d, theta_d, psi_dot_d, theta, phi, phi_dot, theta_dot, psi_dot, P, Q, Vz)

    % Gain Constants
    K1_Q =4.2469;
    K2_Q = 1.6;
    K3_Q = 1;
    k2_vz =2.2;
    k3_vz = 0.5;
    k2_psi = 1.2;
    k3_psi = 0.5;
    K1_P =4.2469;
    K2_P = 1.6;
    K3_P =1;

    % Error Calculation
    Error1 = [(phi_d - phi);
        (theta_d - theta);
              (psi_dot_d - (k2_psi * psi_dot));
              (Vz_d - (k2_vz*Vz))];

    % First Gain Matrix
    Gain_1 = [K1_P  0   0   0;
              0   K1_Q  0   0;
              0   0   k3_psi  0;
              0   0   0   k3_vz];

    % Compute x_dot
    x_dot = Gain_1 * Error1;

    % Extract values
    r_dot_req  = x_dot(3);
    vz_dot_req = x_dot(4);

    % Compute Desired P and Q
    Q_d = (x_dot(2) - (K2_Q * theta_dot));
    P_d = (x_dot(1) - (K2_P * phi_dot));

    % Second Error Calculation
    Error2 = [(P_d - P);
              (Q_d - Q)];

    % Second Gain Matrix
    Gain2 = [K3_P  0;
             0   K3_Q];

    % Compute x_ddot
    x_ddot = Gain2 * Error2;
    % Extract values
    q_dot_req = x_ddot(2);
    P_dot_req = x_ddot(1);

end

== matlab function INDI_QUAD_2021a/Quadrotor/Rotation EqOM Function ==
  data: T1 input; p_dot output; T2 input; T3 input; T4 input; p input; q input; r input; q_dot output; r_dot output; time input; FLT input
function [p_dot,q_dot,r_dot] = fcn(T1,T2,T3,T4,p,q,r,time,FLT)
kt = 66.34;
kq = 2.3114;

l = 1.83/2;
Ix = 0.4688;
Iy = 0.7639;
Iz = 0.4930;
g = 9.81;
    if (time >7.5)
        fault = FLT;
    else
        fault = 1;
    end

    gx = [fault*(-l*kt)/Ix,(l*kt)/Ix,(l*kt)/Ix,(-l*kt)/Ix;
        fault*(l*kt)/Iy,-(l*kt)/Iy,(l*kt)/Iy,-(l*kt)/Iy;
        fault*(kq)/Iz,(kq)/Iz,-(kq)/Iz,-(kq)/Iz;];
    
    tx = [T1;T2;T3;T4];
    
    fx = [-q*r*((Iz-Iy)/Ix); -p*r*((Ix-Iz)/Iy); -p*q*((Iy-Ix)/Iz)];

    
    accel = gx*tx+fx;
    
    p_dot = accel(1);
    q_dot = accel(2);
    r_dot = accel(3);
